simulink model "pendolofeed"  (Simulink 3.00)
settings: Solver=ode23  StartTime=0.0  StopTime=20  MaxStep=0.01  RelTol=1e-9
libraries: simulink3 x1
settings Model: SaveTime=off  SaveOutput=off  UnconnectedInputMsg=none  UnconnectedOutputMsg=none  UnconnectedLineMsg=none  InheritedTsInSrcMsg=none  LastModifiedBy=Administrator

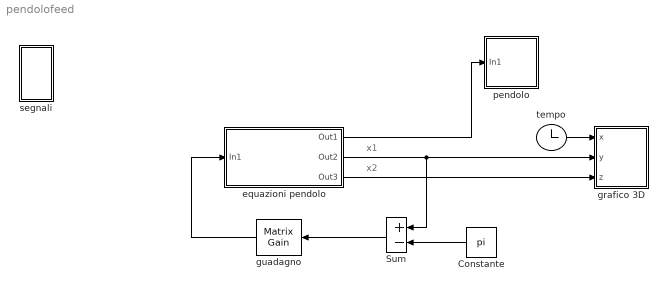
== system pendolofeed ==
  note: x1
  note: x2
  Constante : Constant  Orientation=left  Value=pi
  Sum : Sum  Orientation=left  Inputs=+-  SaturateOnIntegerOverflow=off
  equazioni pendolo : Subsystem  mask(pendolo){x1=pi, x2=0.1}
      mask prompts: x1 "condizione iniziale per x1"; x2 "condizione iniziale per x2"
      mask help:
      | Equazioni che descrizono il moto del pendolo.
      | Introdurre la condizione iniziale per la posizione angolare (x1) in rad
      | e la velocita' angolare (x2) in rad/sec
      mask Display: disp('dx1/dt = x2               \n dx2/dt = -sen(x1)-x2-u')
  grafico 3D : Subsystem  mask(grafico 3D){xlim=[0,20], ylim=[-pi 2*pi], zlim=[-3 3], view=[10 30]}
      mask prompts: xlim "t [min,max]:"; ylim "x1 [min,max]:"; zlim "x2 [min,max]:"; view "orientamento:"
      mask help:
      | Movimento dello stato del sistema
      | Introdurre gli intervalli di rappresentazione del tempo e dello stato
      mask init:
      | st=-1;
      mask Help: This block can be used to explore limit cycles. Look at the m-file sfunxyz.m to see how it works.
      mask Display: plot(0,0,100,100,[12,91,91,12,12],[90,90,45,45,90],[51,57,65,75,80,79,75,67,60,54,51,48,42,34,28,27,31,42,51],[71,68,66,66,72,79,83,84,81,77,71,60,54,54,58,65,71,74,71])
  guadagno : simulink3/Math/Matrix Gain  Orientation=left  K=2
  pendolo : Subsystem  mask(Animation Block){ts=0.05}
      mask prompts: ts "Sample time:"
      mask help: Animazione di un pendolo sottoposto all'azione di una forza
      mask Display: plot([.1,.9],[.9,.9],[.5,.2],[.9,.25],[.475,.475,.525,.525,.475],[.875,.925,.925,.875,.875])
  segnali : Subsystem
  tempo : Clock
      settings: DisplayTime=off  Decimation=10
  wires:
  equazioni pendolo/1(Out1) -> pendolo/1(In1)
  equazioni pendolo/2(Out2) -> grafico 3D/2(y), Sum/1
  tempo/1 -> grafico 3D/1(x)
  equazioni pendolo/3(Out3) -> grafico 3D/3(z)
  guadagno/1 -> equazioni pendolo/1(In1)
  Constante/1 -> Sum/2
  Sum/1 -> guadagno/1

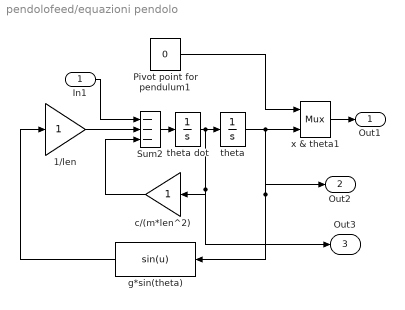
== system pendolofeed/equazioni pendolo ==
  In1 : Inport  Port=1  PortWidth=-1  SampleTime=-1  DataType=auto
      settings: SignalType=auto
  1/len : Gain  Gain=1  SaturateOnIntegerOverflow=on
  Pivot point for pendulum1 : Constant  Value=0
  Sum2 : Sum  Inputs=---  SaturateOnIntegerOverflow=off
  c/(m*len^2) : Gain  Orientation=left  Gain=1  SaturateOnIntegerOverflow=on
  g*sin(theta) : Fcn  Orientation=left  Expr=sin(u)
  theta : Integrator  ExternalReset=none  InitialConditionSource=internal  InitialCondition=x1  LimitOutput=off  UpperSaturationLimit=inf  LowerSaturationLimit=-inf  ShowSaturationPort=off  ShowStatePort=off  AbsoluteTolerance=auto
  theta dot : Integrator  ExternalReset=none  InitialConditionSource=internal  InitialCondition=x2  LimitOutput=off  UpperSaturationLimit=inf  LowerSaturationLimit=-inf  ShowSaturationPort=off  ShowStatePort=off  AbsoluteTolerance=auto
  x & theta1 : Mux  Inputs=2
      settings: DisplayOption=none
  Out1 : Outport  Port=1
  Out2 : Outport  Port=2
  Out3 : Outport  Port=3
  wires:
  Sum2/1 -> theta dot/1
  c/(m*len^2)/1 -> Sum2/3
  theta dot/1 -> theta/1, c/(m*len^2)/1, Out3/1
  Pivot point for pendulum1/1 -> x & theta1/1
  theta/1 -> x & theta1/2, g*sin(theta)/1, Out2/1
  1/len/1 -> Sum2/2
  g*sin(theta)/1 -> 1/len/1
  x & theta1/1 -> Out1/1
  In1/1 -> Sum2/1

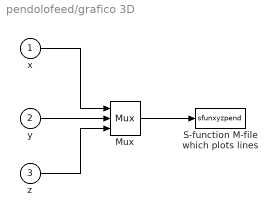
== system pendolofeed/grafico 3D ==
  x : Inport  Port=1  PortWidth=-1  SampleTime=-1  DataType=auto
      settings: SignalType=auto
  y : Inport  Port=2  PortWidth=-1  SampleTime=-1  DataType=auto
      settings: SignalType=auto
  z : Inport  Port=3  PortWidth=-1  SampleTime=-1  DataType=auto
      settings: SignalType=auto
  Mux : Mux  Inputs=3
      settings: DisplayOption=none
  "S-function M-file which plots lines " : S-Function  FunctionName=sfunxyzpend  Parameters=xlim,ylim,zlim,view,st  PortCounts=[]  SFunctionModules=''
  wires:
  z/1 -> Mux/3
  y/1 -> Mux/2
  x/1 -> Mux/1
  Mux/1 -> "S-function M-file which plots lines "/1

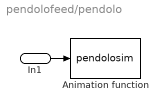
== system pendolofeed/pendolo ==
  In1 : Inport  Port=1  PortWidth=-1  SampleTime=-1  DataType=auto
      settings: SignalType=auto
  Animation function : S-Function  FunctionName=pendolosim  Parameters=ts  PortCounts=[]  SFunctionModules=''
      settings: DeleteFcn=if ~isempty(findobj('type','figure','name','simppend Animation'));close('simppend Animation'); end;
  wires:
  In1/1 -> Animation function/1

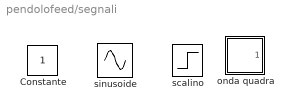
== system pendolofeed/segnali ==
  Constante : Constant  Value=1
  onda quadra : Subsystem  mask(Pulse Generator){@1=2, @2=1, @3=1, @4=0}
      mask prompts: @1 "Pulse period (secs):"; @2 "Pulse width:"; @3 "Pulse height:"; @4 "Pulse start time:"
      mask help: Pulse Generator.
      mask init:
      | Ts=@1; du=@2; ht=@3; stt=@4; ini=ones(length(ht),1); st1=rem(stt,Ts); st2=rem(stt+du,Ts);if(Ts<=1.2*du),ini=zeros(length(ht),1);end;
      mask Help: Pulse generator which ensures pulse\ntransitions are hit. Provides a vector of pulses when the height is entered as a vector.\nUnmask to see how it works.
      mask Display: plot(0,0,100,100,[90,75,75,60,60,35,35,20,20,10],[20,20,80,80,20,20,80,80,20,20])
  scalino : Step  Time=0  Before=0  After=1  SampleTime=-1
  sinusoide : Sin  Amplitude=1  Frequency=1  Phase=0  SampleTime=-1

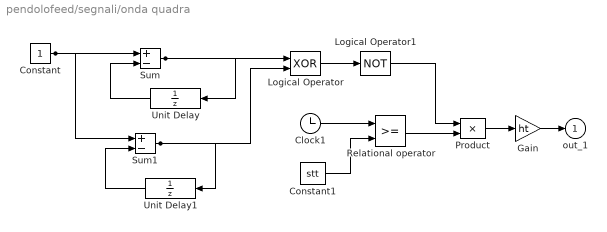
== system pendolofeed/segnali/onda quadra ==
  Clock1 : Clock
      settings: DisplayTime=off  Decimation=10
  Constant : Constant  Value=1
  Constant1 : Constant  Value=stt
  Gain : Gain  Gain=ht  SaturateOnIntegerOverflow=on
  Logical Operator : Logic  Operator=XOR  Inputs=2
  Logical Operator1 : Logic  Operator=NOT  Inputs=1
  Product : Product  Inputs=2  SaturateOnIntegerOverflow=on
  Relational operator : RelationalOperator  Operator=>=
  Sum : Sum  Inputs=+-  SaturateOnIntegerOverflow=on
  Sum1 : Sum  Inputs=+-  SaturateOnIntegerOverflow=on
  Unit Delay : UnitDelay  Orientation=left  X0=0  SampleTime=[Ts,st1]
  Unit Delay1 : UnitDelay  Orientation=left  X0=ini  SampleTime=[Ts,st2]
  out_1 : Outport  Port=1
  wires:
  Logical Operator1/1 -> Product/1
  Logical Operator/1 -> Logical Operator1/1
  Constant1/1 -> Relational operator/2
  Gain/1 -> out_1/1
  Product/1 -> Gain/1
  Relational operator/1 -> Product/2
  Clock1/1 -> Relational operator/1
  Unit Delay/1 -> Sum/2
  Unit Delay1/1 -> Sum1/2
  Constant/1 -> Sum/1, Sum1/1
  Sum/1 -> Unit Delay/1, Logical Operator/1
  Sum1/1 -> Unit Delay1/1, Logical Operator/2
